simulink model "sampleModel1841"  (R2023a)
settings: Solver=VariableStepAuto  StartTime=0.0  StopTime=10.0  RelTol=1e-3
libraries: hdlsllib x8, simulink x3
settings Model: Creator=user1  LastModifiedBy=user1

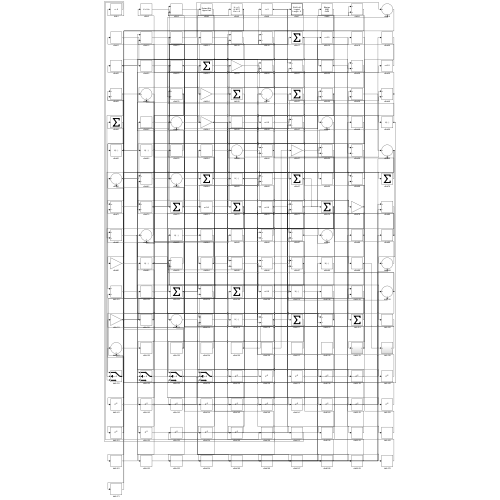
[thumbnail: Simulink's stored preview of the top-level diagram]
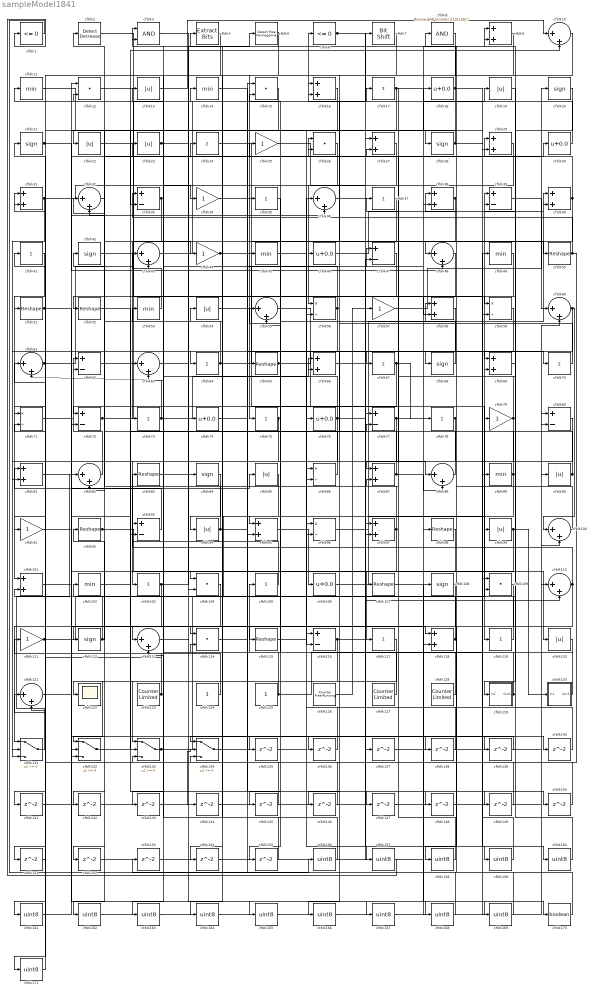
== system sampleModel1841 ==
  cfblk1 : hdlsllib/Logic and Bit Operations/Compare To Zero  relop=<=  OutDataTypeStr=boolean
  cfblk{10,32,36,43,48,55,60..61,63,82,88,100,110,113,121} (15 alike) : Sum  Inputs=|++
  cfblk{9,16,27,29,31,38,40,58,66,69,81,87,95,97,101,118} (16 alike) : Sum
  cfblk{11,14,45,49,53,89,102} (7 alike) : MinMax
  cfblk{17,24,35,37,41,64,67,70,73,75,78,103,105,117,119} (15 alike) : Sum  Inputs=+
  cfblk{12,15,26,104,109,114} (6 alike) : DotProduct  OutDataTypeStr=Inherit: Inherit via internal rule
  cfblk{18,30,46,74,76,106} (6 alike) : Bias  Bias=0.0  SaturateOnIntegerOverflow=off
  cfblk{50..52,65,83,92,98,107,115} (9 alike) : Reshape
  cfblk{20..21,28,42,68,84,108,112} (8 alike) : Signum
  cfblk{25,34,44,57,79,91,111} (7 alike) : Gain
  cfblk{33,39,47,62,72,77,80,93,116} (9 alike) : Sum  Inputs=+-
  cfblk{13,19,22..23,54,85,90,94,99,120} (10 alike) : Abs  SaturateOnIntegerOverflow=off
  cfblk122 : Scope
  cfblk123 : hdlsllib/Sources/Counter Limited  uplimit=7  tsamp=-1
  cfblk124 : Constant  SampleTime=-1
  cfblk125 : Constant  SampleTime=-1
  cfblk126 : hdlsllib/Sources/Counter Free-Running  NumBits=16  tsamp=-1
  cfblk127 : hdlsllib/Sources/Counter Limited  uplimit=7  tsamp=-1
  cfblk128 : hdlsllib/Sources/Counter Limited  uplimit=7  tsamp=-1
  cfblk129 : Subsystem
      settings: LibrarySourceBlock=|
      | hdlsllib/Ports &
      | Subsystems/Subsystem
  cfblk130 : Subsystem
      settings: LibrarySourceBlock=|
      | hdlsllib/Ports &
      | Subsystems/Subsystem
  cfblk{131..134} (4 alike) : Switch  SaturateOnIntegerOverflow=off  InputSameDT=off
  cfblk{135..155} (21 alike) : Delay  SampleTime=1
  cfblk{156..169,171} (15 alike) : DataTypeConversion  OutDataTypeStr=uint8  SaturateOnIntegerOverflow=off  RndMeth=Floor
  cfblk170 : DataTypeConversion  OutDataTypeStr=boolean  SaturateOnIntegerOverflow=off  RndMeth=Floor
  cfblk2 : simulink/Logic and Bit Operations/Detect Decrease  vinit=0.0  OutDataTypeStr=boolean
      settings: LibrarySourceBlock=|
      | hdlsllib/Logic and Bit
      | Operations/Detect
      | Decrease
  cfblk3 : Logic  AllPortsSameDT=off  OutDataTypeStr=boolean
  cfblk4 : simulink/Logic and Bit Operations/Extract Bits  bitsToExtract=Upper half  numBits=8  bitIdxRange=[0 7]  outScalingMode=Preserve fixed-point scaling
      settings: LibrarySourceBlock=|
      | hdlsllib/Logic and Bit
      | Operations/Extract Bits
  cfblk5 : hdlsllib/Logic and Bit Operations/Detect Rise Nonnegative  vinit=0  OutDataTypeStr=boolean
  cfblk{56,59,71,86,96} (5 alike) : Product  Inputs=*/  RndMeth=Zero  SaturateOnIntegerOverflow=on
  cfblk6 : hdlsllib/Logic and Bit Operations/Compare To Zero  relop=<=  OutDataTypeStr=boolean
  cfblk7 : hdlsllib/Logic and Bit Operations/Bit Shift  mode=Shift Left Logical  N=0
  cfblk8 : simulink/Logic and Bit Operations/Bitwise Operator  logicop=AND  UseBitMask=on  BitMask=bin2dec('11011001')  BitMaskRealWorld=Stored Integer
      settings: LibrarySourceBlock=|
      | hdlsllib/Logic and Bit
      | Operations/Bitwise
      | Operator
  wires:
  cfblk72/1 -> cfblk14/1, cfblk30/1
  cfblk7/1 -> cfblk104/1
  cfblk13/1 -> cfblk10/1
  cfblk126/1 -> cfblk57/1
  cfblk78/1 -> cfblk103/1, cfblk145/1, cfblk146/1
  cfblk41/1 -> cfblk101/1
  cfblk106/1 -> cfblk40/1
  cfblk5/1 -> cfblk75/1, cfblk71/1
  cfblk42/1 -> cfblk17/1
  cfblk34/1 -> cfblk119/1
  cfblk85/1 -> cfblk102/1
  cfblk24/1 -> cfblk50/1
  cfblk43/1 -> cfblk7/1
  cfblk60/1 -> cfblk100/1, cfblk72/2, cfblk81/2
  cfblk133/1 -> cfblk45/1, cfblk147/1
  cfblk111/1 -> cfblk39/1, cfblk65/1
  cfblk97/1 -> cfblk42/1, cfblk133/2, cfblk132/3
  cfblk33/1 -> cfblk73/1, cfblk152/1
  cfblk29/1 -> cfblk56/1
  cfblk100/1 -> cfblk25/1
  cfblk20/1 -> cfblk59/1
  cfblk31/1 -> cfblk34/1, cfblk131/3
  cfblk47/1 -> cfblk95/1
  cfblk18/1 -> cfblk3/1, cfblk33/2, cfblk160/1
  cfblk23/1 -> cfblk84/1, cfblk63/1
  cfblk17/1 -> cfblk87/1, cfblk29/2, cfblk91/1
  cfblk22/1 -> cfblk44/1
  cfblk46/1 -> cfblk40/2
  cfblk38/1 -> cfblk48/1, cfblk72/1
  cfblk12/1 -> cfblk59/2
  cfblk44/1 -> cfblk58/2, cfblk150/1
  cfblk131/1 -> cfblk82/1
  cfblk76/1 -> cfblk114/1, cfblk3/2, cfblk110/2, cfblk95/2
  cfblk30/1 -> cfblk6/1
  cfblk127/1 -> cfblk105/1
  cfblk115/1 -> cfblk36/1
  cfblk55/1 -> cfblk79/1
  cfblk103/1 -> cfblk131/1, cfblk5/1, cfblk26/2
  cfblk89/1 -> cfblk15/2, cfblk155/1
  cfblk96/1 -> cfblk99/1
  cfblk57/1 -> cfblk20/1
  cfblk61/1 -> cfblk16/1, cfblk118/2
  cfblk65/1 -> cfblk69/1, cfblk118/1
  cfblk124/1 -> cfblk111/1
  cfblk93/1 -> cfblk81/1
  cfblk69/1 -> cfblk9/1
  cfblk99/1 -> cfblk117/1, cfblk130/1(In1)
  cfblk40/1 -> cfblk64/1, cfblk2/1
  cfblk94/1 -> cfblk66/1, cfblk32/1
  cfblk116/1 -> cfblk133/1, cfblk148/1
  cfblk110/1 -> cfblk83/1, cfblk58/1, cfblk154/1
  cfblk123/1 -> cfblk41/1, cfblk71/2
  cfblk37/1 -> cfblk56/2
  cfblk62/1 -> cfblk48/2
  cfblk82/1 -> cfblk62/1
  cfblk14/1 -> cfblk68/1
  cfblk86/1 -> cfblk23/1
  cfblk119/1 -> cfblk101/2
  cfblk32/1 -> cfblk52/1
  cfblk6/1 -> cfblk27/1, cfblk159/1
  cfblk28/1 -> cfblk22/1, cfblk70/1
  cfblk49/1 -> cfblk122/1
  cfblk73/1 -> cfblk66/2, cfblk61/2
  cfblk92/1 -> cfblk120/1, cfblk116/2, cfblk149/1
  cfblk10/1 -> cfblk113/1
  cfblk125/1 -> cfblk49/1, cfblk13/1
  cfblk11/1 -> cfblk116/1
  cfblk101/1 -> cfblk29/1
  cfblk79/1 -> cfblk27/2, cfblk96/2
  cfblk64/1 -> cfblk18/1, cfblk32/2
  cfblk70/1 -> cfblk26/1
  cfblk75/1 -> cfblk104/2, cfblk131/2
  cfblk83/1 -> cfblk74/1
  cfblk9/1 -> cfblk46/1
  cfblk112/1 -> cfblk92/1, cfblk21/1
  cfblk68/1 -> cfblk24/1
  cfblk91/1 -> cfblk85/1
  cfblk120/1 -> cfblk114/2
  cfblk54/1 -> cfblk19/1
  cfblk39/1 -> cfblk60/1
  cfblk45/1 -> cfblk67/1
  cfblk4/1 -> cfblk51/1
  cfblk128/1 -> cfblk53/1
  cfblk27/1 -> cfblk35/1
  cfblk129/1(Out1) -> cfblk39/2, cfblk55/2
  cfblk71/1 -> cfblk62/2
  cfblk87/1 -> cfblk55/1, cfblk88/2
  cfblk67/1 -> cfblk78/1, cfblk142/1
  cfblk53/1 -> cfblk43/1
  cfblk25/1 -> cfblk97/2
  cfblk51/1 -> cfblk36/2, cfblk93/2, cfblk31/1
  cfblk19/1 -> cfblk129/1(In1)
  cfblk77/1 -> cfblk86/2, cfblk9/2
  cfblk2/1 -> cfblk107/1
  cfblk88/1 -> cfblk16/2
  cfblk118/1 -> cfblk4/1, cfblk112/1
  cfblk105/1 -> cfblk93/1
  cfblk56/1 -> cfblk11/1, cfblk141/1
  cfblk74/1 -> cfblk47/1
  cfblk132/1 -> cfblk77/2
  cfblk16/1 -> cfblk82/2
  cfblk90/1 -> cfblk38/1, cfblk12/2
  cfblk84/1 -> cfblk94/1
  cfblk26/1 -> cfblk113/2
  cfblk52/1 -> cfblk115/1
  cfblk134/1 -> cfblk76/1
  cfblk95/1 -> cfblk106/1
  cfblk130/1(Out1) -> cfblk69/2
  cfblk117/1 -> cfblk132/1
  cfblk66/1 -> cfblk88/1
  cfblk102/1 -> cfblk10/2
  cfblk50/1 -> cfblk134/3, cfblk33/1
  cfblk21/1 -> cfblk28/1, cfblk43/2
  cfblk35/1 -> cfblk135/1
  cfblk59/1 -> cfblk136/1
  cfblk136/1 -> cfblk86/1
  cfblk36/1 -> cfblk137/1
  cfblk137/1 -> cfblk60/2
  cfblk114/1 -> cfblk138/1
  cfblk138/1 -> cfblk77/1
  cfblk3/1 -> cfblk139/1
  cfblk139/1 -> cfblk134/1
  cfblk81/1 -> cfblk140/1
  cfblk140/1 -> cfblk96/1
  cfblk141/1 -> cfblk134/2
  cfblk142/1 -> cfblk97/1
  cfblk104/1 -> cfblk143/1
  cfblk113/1 -> cfblk144/1
  cfblk144/1 -> cfblk100/2
  cfblk145/1 -> cfblk133/3
  cfblk146/1 -> cfblk31/2
  cfblk147/1 -> cfblk87/2
  cfblk148/1 -> cfblk110/1
  cfblk149/1 -> cfblk132/2
  cfblk150/1 -> cfblk61/1
  cfblk58/1 -> cfblk151/1
  cfblk151/1 -> cfblk121/2
  cfblk152/1 -> cfblk47/2
  cfblk154/1 -> cfblk38/2
  cfblk155/1 -> cfblk63/2
  cfblk1/1 -> cfblk156/1
  cfblk156/1 -> cfblk54/1
  cfblk135/1 -> cfblk157/1
  cfblk157/1 -> cfblk1/1
  cfblk109/1 -> cfblk158/1
  cfblk158/1 -> cfblk37/1
  cfblk159/1 -> cfblk109/1
  cfblk160/1 -> cfblk109/2
  cfblk108/1 -> cfblk161/1
  cfblk161/1 -> cfblk12/1
  cfblk48/1 -> cfblk162/1
  cfblk162/1 -> cfblk108/1
  cfblk80/1 -> cfblk163/1
  cfblk163/1 -> cfblk90/1
  cfblk15/1 -> cfblk164/1
  cfblk164/1 -> cfblk80/1
  cfblk143/1 -> cfblk165/1
  cfblk165/1 -> cfblk80/2
  cfblk98/1 -> cfblk166/1
  cfblk166/1 -> cfblk89/1
  cfblk121/1 -> cfblk167/1
  cfblk167/1 -> cfblk98/1
  cfblk153/1 -> cfblk168/1
  cfblk168/1 -> cfblk15/1
  cfblk107/1 -> cfblk169/1
  cfblk169/1 -> cfblk153/1
  cfblk63/1 -> cfblk170/1
  cfblk170/1 -> cfblk8/1
  cfblk8/1 -> cfblk171/1
  cfblk171/1 -> cfblk121/1

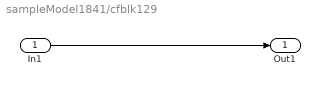
== system sampleModel1841/cfblk129 ==
  In1 : Inport
  Out1 : Outport
  wires:
  In1/1 -> Out1/1

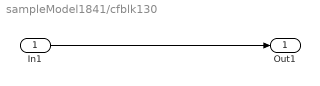
== system sampleModel1841/cfblk130 ==
  In1 : Inport
  Out1 : Outport
  wires:
  In1/1 -> Out1/1
